simulink model "px4demo_HostSerial_TxRx20190112"  (R2016b)
settings: Solver=VariableStepAuto  StartTime=0.0  StopTime=inf  RelTol=1e-3  EnableMultiTasking=on
undefined symbols (not defined in the file or in its folder): serial
libraries: instrumentlib x3, aerolibanimutils x1
settings Model: Creator=darenlee  LastModifiedBy=E6320
settings DataIOCC: LimitDataPoints=on
settings OptimizationCC: LifeSpan=inf
settings DebuggingCC: ParameterOverflowMsg=none  AllowSymbolicDim=off  SFUnexpectedBacktrackingDiag=warning  SFNoUnconditionalDefaultTransitionDiag=warning  SFExecutionAtInitializationDiag=none
settings ModelReferenceCC: PropagateSignalLabelsOutOfModel=off
settings GRTTargetCC: TargetLangStandard=C89/C90 (ANSI)
settings ConfigComp: CovMetricSettings=dw  CovHtmlReporting=on  CovSaveCumulativeToWorkspaceVar=on  CovSaveSingleToWorkspaceVar=on  CovExternalEMLEnable=off

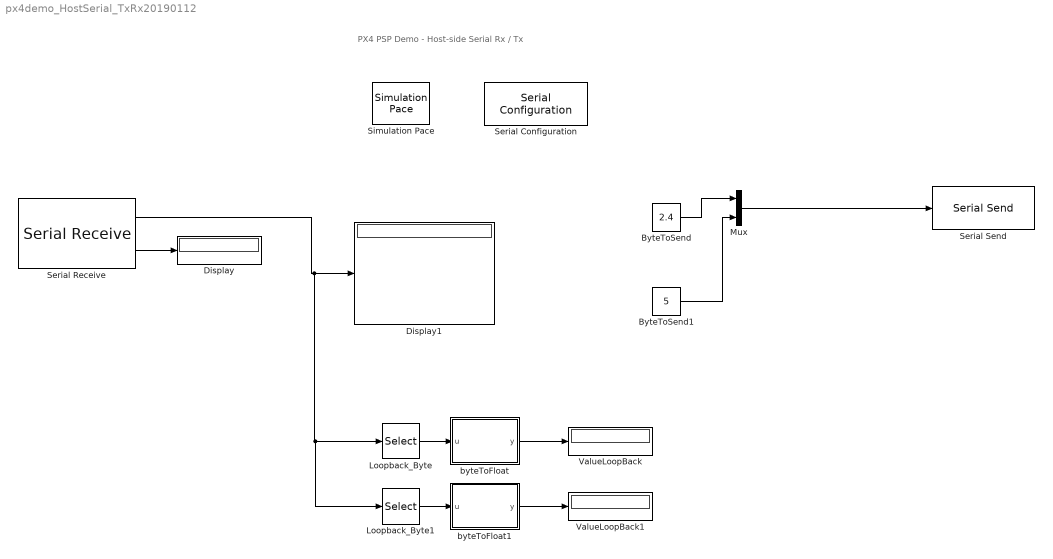
== system px4demo_HostSerial_TxRx20190112 ==
  note: PX4 PSP Demo - Host-side Serial Rx / Tx
  ByteToSend : Constant  Value=2.4  VectorParams1D=off  OutDataTypeStr=uint8  SampleTime=0.005
  ByteToSend1 : Constant  Value=5  VectorParams1D=off  OutDataTypeStr=uint8  SampleTime=0.005
  Display : Display
  Display1 : Display
  Loopback_Byte : Selector  InputPortWidth=8  IndexOptions=Index vector (dialog)  Indices=1:4  OutputSizes=1
  Loopback_Byte1 : Selector  InputPortWidth=8  IndexOptions=Index vector (dialog)  Indices=5:8  OutputSizes=1
  Mux : Mux  Inputs=2
  Serial Configuration : instrumentlib/Serial Configuration  Priority=-200000  ComPortMenu=COM10  ComPort=COM10  ObjConstructor=serial('COM10');  BaudRate=57600  DataBits=8  Parity=none  StopBits=1  FlowControl=none  Timeout=10  ByteOrder=LittleEndian
  Serial Receive : instrumentlib/Serial Receive  ComPortMenu=COM10  ComPort=COM10  ObjConstructor=serial('COM10');  Terminator=<none>  DataSize="[8  1]"  DataType=uint8  EnableBlockingMode=off  ActionDataUnavailable=Output last received value  CustomValue=0  SampleTime=0.5
  Serial Send : instrumentlib/Serial Send  ComPortMenu=COM10  ComPort=COM10  ObjConstructor=serial('COM10');  Terminator=<none>  EnableBlockingMode=off
  Simulation Pace : aerolibanimutils/Simulation Pace  SimulationPace=1  SleepMode=MATLAB Thread  OutputPaceError=off  SampleTime=0.5
  ValueLoopBack : Display
  ValueLoopBack1 : Display
  byteToFloat : MATLAB Function  TreatAsAtomicUnit=on
  byteToFloat1 : MATLAB Function  TreatAsAtomicUnit=on
  wires:
  Loopback_Byte/1 -> byteToFloat/1(u)
  byteToFloat/1(y) -> ValueLoopBack/1
  Serial Receive/2 -> Display/1
  Loopback_Byte1/1 -> byteToFloat1/1(u)
  byteToFloat1/1(y) -> ValueLoopBack1/1
  Mux/1 -> Serial Send/1
  Serial Receive/1 -> Loopback_Byte1/1, Loopback_Byte/1, Display1/1
  ByteToSend1/1 -> Mux/2
  ByteToSend/1 -> Mux/1

== matlab function px4demo_HostSerial_TxRx20190112/byteToFloat1 ==
  data: u input; y output
function y = fcn(u)
%#codegen
y = single(0);
y = single(typecast(uint8(u),'single'));
% y = u;

== matlab function px4demo_HostSerial_TxRx20190112/byteToFloat ==
  data: u input; y output
function y = fcn(u)
%#codegen
y = single(0);
y = single(typecast(uint8(u),'single'));
% y = u;
